simulink library "LeftIndicator"  (R2015a)
settings: Solver=ode45  StartTime=0.0  StopTime=10.0  RelTol=1e-3
settings Model: Creator=Bruno  LastModifiedBy=Bruno

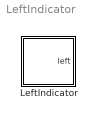
== system LeftIndicator ==
  LeftIndicator : Stateflow chart  TreatAsAtomicUnit=on

== stateflow chart LeftIndicator/LeftIndicator ==
  state Off
    entry:
    left=0
    during: delay(10)
  state On
    entry:
    left=1
    during: delay(10)
  On -> Off
  (default) -> Off
  Off -> On
  data: left output double size=1
